simulink model "nois"  (R2020b)
settings: Solver=VariableStepAuto  StartTime=0.0  StopTime=150  RelTol=1e-3
values from neighbouring files (symbols this model uses):
  Ts = 0.1    [all_signals.m]    (also in cutting_signals.m; get_outputs.m; main_3.m; noise.m)
libraries: PoKeysIOInterface x1
settings Model: Creator=64170108  LastModifiedBy=64170108

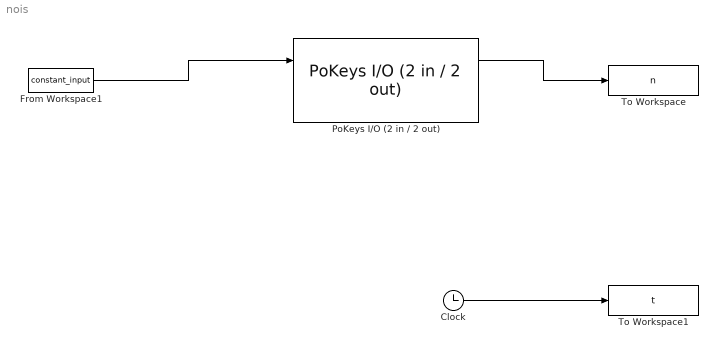
== system nois ==
  Clock : Clock
  From Workspace1 : FromWorkspace  VariableName=constant_input  SampleTime=Ts
  PoKeys I/O (2 in / 2 out) : PoKeysIOInterface/PoKeys I//O (2 in // 2 out)  MaxPowerLimit=100.0  IOTs=Ts  IOSerial=500
      settings: SourceProductName=PoKeys I/O interface
  To Workspace : ToWorkspace  VariableName=n  SampleTime=Ts
  To Workspace1 : ToWorkspace  VariableName=t  SampleTime=Ts
  wires:
  Clock/1 -> To Workspace1/1
  PoKeys I/O (2 in / 2 out)/1 -> To Workspace/1
  From Workspace1/1 -> PoKeys I/O (2 in / 2 out)/1
